simulink model "fouriersimu"  (R2016a)
settings: Solver=VariableStepAuto  StartTime=0.0  StopTime=10.0  RelTol=1e-3
settings Model: Creator=iP Store  LastModifiedBy=iP Store

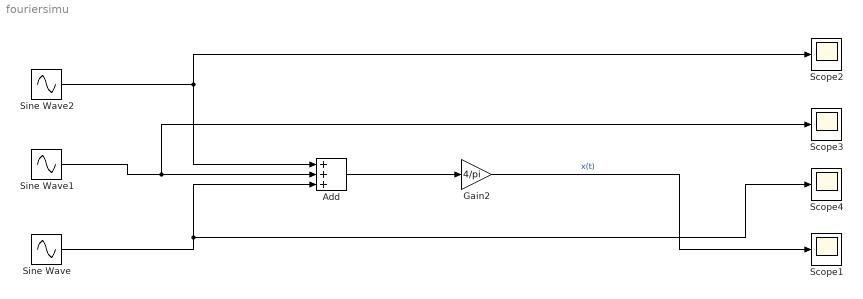
== system fouriersimu ==
  Add : Sum  Inputs=+++
  Gain2 : Gain  Gain=4/pi
  Scope{1..4} (4 alike) : Scope
  Sine Wave : Sin  SampleTime=0
  Sine Wave1 : Sin  Amplitude=1/3  Frequency=3  SampleTime=0
  Sine Wave2 : Sin  Amplitude=1/5  Frequency=5  SampleTime=0
  wires:
  Sine Wave/1 -> Scope4/1, Add/3
  Add/1 -> Gain2/1
  Sine Wave1/1 -> Scope3/1, Add/2
  Sine Wave2/1 -> Scope2/1, Add/1
  Gain2/1 -> Scope1/1  "x(t)"
